simulink model "EV_lunwen_mohu"  (R2018a)
settings: Solver=VariableStepAuto  StartTime=0.0  StopTime=1370  RelTol=1e-3
undefined symbols (not defined in the file or in its folder): batt, cyc_spd, cyc_time, DiscIntNeverNeededParam, fr_effi, TIME_STEP, tm, UC, vcu, vehicle
libraries: simulink x10, fuzblock x1
(part 2 of 2)

== system EV_lunwen_mohu/Vehicle/Fj ==
  veh_spd_mps : Inport
  Dead Zone : DeadZone  LowerValue=-0.01  UpperValue=0.01  SaturateOnIntegerOverflow=on
  Discrete Derivative : simulink/Discrete/Discrete Derivative  gainval=1.0  ICPrevScaledInput=0.0  InputProcessing=Inherited  OutMin=[]  OutMax=[]  OutDataType=fixdt(1, 16)  OutScaling=2^-10  DoSatur=off
  Product1 : Product  SaturateOnIntegerOverflow=on  InputSameDT=on  OutDataTypeStr=Inherit: Same as first input
  Product4 : Product  Inputs=3
  m : Constant  Value=vehicle.veh_mass_kg
  sign(u) : Lookup  InputValues=[ -0.1 0.1 ]  Table="[-1  1]"  LookUpMeth=Interpolation-Use End Values  OutDataTypeStr=double  SaturateOnIntegerOverflow=on
  旋转质量换算系数 : Constant
  Fj : Outport  InitialOutput=0
  wires:
  veh_spd_mps/1 -> Dead Zone/1, Discrete Derivative/1
  Discrete Derivative/1 -> Product4/2
  旋转质量换算系数/1 -> Product4/3
  m/1 -> Product4/1
  sign(u)/1 -> Product1/1
  Dead Zone/1 -> sign(u)/1
  Product4/1 -> Product1/2
  Product1/1 -> Fj/1

== system EV_lunwen_mohu/Vehicle/Fw ==
  veh_spd_mps : Inport
  Dead Zone : DeadZone  LowerValue=-0.01  UpperValue=0.01  SaturateOnIntegerOverflow=on
  Dead Zone1 : DeadZone  LowerValue=-0.01  UpperValue=0.01  SaturateOnIntegerOverflow=on
  Product1 : Product  SaturateOnIntegerOverflow=on  InputSameDT=on  OutDataTypeStr=Inherit: Same as first input
  Product2 : Product  SaturateOnIntegerOverflow=on  InputSameDT=on  OutDataTypeStr=Inherit: Same as first input
  Wind Resistane : Gain  Gain=0.5*vehicle.air_density_kgpm3*vehicle.Cd*vehicle.veh_fac_area_m2  SaturateOnIntegerOverflow=on  OutDataTypeStr=Inherit: Same as input  ParamDataTypeStr=Inherit: Same as input
  sign(u) : Lookup  InputValues=[ -0.1 0.1 ]  Table="[-1  1]"  LookUpMeth=Interpolation-Use End Values  OutDataTypeStr=double  SaturateOnIntegerOverflow=on
  Fi : Outport  InitialOutput=0
  wires:
  Product1/1 -> Wind Resistane/1
  veh_spd_mps/1 -> Dead Zone1/1, Dead Zone/1
  Dead Zone/1 -> Product1/2, Product1/1
  sign(u)/1 -> Product2/1
  Dead Zone1/1 -> sign(u)/1
  Wind Resistane/1 -> Product2/2
  Product2/1 -> Fi/1

== system EV_lunwen_mohu/Vehicle/inertia ==
  inertia_in : Inport
  Product6 : Product  Inputs=3  OutDataTypeStr=double  SaturateOnIntegerOverflow=on  InputSameDT=on
  Sum2 : Sum  Inputs=+++  OutDataTypeStr=double  SaturateOnIntegerOverflow=on
  Tyre radius (m) : Constant  Value=vehicle.tyre_radius_m
  Tyre radius (m)1 : Constant  Value=vehicle.tyre_inertia
  Vehicle mass (kg) : Constant  Value=vehicle.veh_mass_kg
  rad/s^2 to m/s^2 1 : Gain  Gain=4  SaturateOnIntegerOverflow=on  OutDataTypeStr=Inherit: Same as input  ParamDataTypeStr=Inherit: Same as input
  rad/s^2 to m/s^2 2 : Gain  Gain=vehicle.fr_ratio * vehicle.fr_ratio  SaturateOnIntegerOverflow=on  OutDataTypeStr=Inherit: Same as input  ParamDataTypeStr=Inherit: Same as input
  Inertia coefficient : Outport  InitialOutput=0
  wires:
  Tyre radius (m)1/1 -> rad/s^2 to m/s^2 1/1
  Tyre radius (m)/1 -> Product6/3, Product6/2
  Vehicle mass (kg)/1 -> Product6/1
  inertia_in/1 -> rad/s^2 to m/s^2 2/1  "tm_Inertia"
  rad/s^2 to m/s^2 2/1 -> Sum2/1
  Product6/1 -> Sum2/2
  rad/s^2 to m/s^2 1/1 -> Sum2/3
  Sum2/1 -> Inertia coefficient/1

== system EV_lunwen_mohu/BATT/max power limitation/peak chrg power ==
  note: 电池电流
  note: 损耗电压
  note: 电池端电压
  batt_res_ohms : Inport
  batt_oc_volt_v : Inport  Port=2
  Constant : Constant  Value=batt.cell_max_volt_v * batt.cells_series_no
  Constant1 : Constant  Value=0
  Divide : Product  Inputs=*/
  Gain1 : Gain  Gain=1/1000
  MinMax1 : MinMax  Inputs=2  SaturateOnIntegerOverflow=on  InputSameDT=on
  Product2 : Product  SaturateOnIntegerOverflow=on  OutDataTypeStr=Inherit: Same as first input
  Sum1 : Sum  Inputs=+-  SaturateOnIntegerOverflow=on  InputSameDT=on  OutDataTypeStr=Inherit: Same as first input
  chrg_peak_pwr_kw : Outport
  wires:
  Gain1/1 -> chrg_peak_pwr_kw/1
  MinMax1/1 -> Gain1/1
  Constant1/1 -> MinMax1/2
  Product2/1 -> MinMax1/1
  Divide/1 -> Product2/1
  batt_res_ohms/1 -> Divide/2
  Sum1/1 -> Divide/1
  Constant/1 -> Product2/2, Sum1/2
  batt_oc_volt_v/1 -> Sum1/1

== system EV_lunwen_mohu/BATT/max power limitation/peak dischrg power ==
  batt_res_ohms : Inport
  batt_oc_volt_v : Inport  Port=2
  Constant : Constant  Value=batt.cell_min_volt_v * batt.cells_series_no
  Constant1 : Constant  Value=0
  Divide : Product  Inputs=*/
  Gain1 : Gain  Gain=1/1000
  MinMax1 : MinMax  Function=max  Inputs=2  SaturateOnIntegerOverflow=on  InputSameDT=on
  Product2 : Product  SaturateOnIntegerOverflow=on  OutDataTypeStr=Inherit: Same as first input
  Sum1 : Sum  Inputs=+-  SaturateOnIntegerOverflow=on  InputSameDT=on  OutDataTypeStr=Inherit: Same as first input
  dischrg_peak_pwr_kw : Outport
  wires:
  Gain1/1 -> dischrg_peak_pwr_kw/1
  MinMax1/1 -> Gain1/1
  Constant1/1 -> MinMax1/2
  Product2/1 -> MinMax1/1
  Divide/1 -> Product2/1
  batt_res_ohms/1 -> Divide/2
  Sum1/1 -> Divide/1
  Constant/1 -> Product2/2, Sum1/2
  batt_oc_volt_v/1 -> Sum1/1

== system EV_lunwen_mohu/UC and dc//dc/UC/Internal Heating ==
  amb_temp_degc : Inport
  Iout : Inport  Port=2
  lost_volt_v : Inport  Port=3
  1/thermal capacity : Gain  Gain=1/(batt.thermal_capa_jpk*UC.ess_parallel_mod_num*UC.ess_module_num)  SaturateOnIntegerOverflow=on  OutDataTypeStr=Inherit: Same as input  ParamDataTypeStr=Inherit: Same as input
  1/thermal resistance : Gain  Gain=batt.thermal_disp_wpk  SaturateOnIntegerOverflow=on  OutDataTypeStr=Inherit: Same as input  ParamDataTypeStr=Inherit: Same as input
  Abs : Abs  SaturateOnIntegerOverflow=on
  Discrete-Time Integrator1 : DiscreteIntegrator  SampleTime=0.01  LimitOutput=on  LowerSaturationLimit=0  ICPrevOutput=DiscIntNeverNeededParam  ICPrevScaledInput=DiscIntNeverNeededParam
  Product1 : Product  SaturateOnIntegerOverflow=on  InputSameDT=on  OutDataTypeStr=Inherit: Same as first input
  Sum1 : Sum  Inputs=+-  SaturateOnIntegerOverflow=on  InputSameDT=on  OutDataTypeStr=Inherit: Same as first input
  Sum2 : Sum  Inputs=+-  SaturateOnIntegerOverflow=on  InputSameDT=on  OutDataTypeStr=Inherit: Same as first input
  To Workspace : ToWorkspace  VariableName=ess_temp_degc  SaveFormat=Timeseries  SampleTime=-1
  ess_temp_degc : Outport  InitialOutput=0
  wires:
  Sum2/1 -> 1/thermal resistance/1
  amb_temp_degc/1 -> Sum2/2
  Product1/1 -> Abs/1
  Abs/1 -> Sum1/1
  Sum1/1 -> 1/thermal capacity/1
  1/thermal resistance/1 -> Sum1/2
  Iout/1 -> Product1/1
  lost_volt_v/1 -> Product1/2
  1/thermal capacity/1 -> Discrete-Time Integrator1/1
  Discrete-Time Integrator1/1 -> To Workspace/1, ess_temp_degc/1, Sum2/1

== system EV_lunwen_mohu/UC and dc//dc/UC/Subsystem ==
  Preq : Inport
  Voc : Inport  Port=2
  tmp : Inport  Port=3
  SOC : Inport  Port=4
  " " : Fcn  Expr=(u(1)/(u(2)+eps))
  -1*|u| : Fcn  Expr=-1*abs(u)
  Abs : Abs  SaturateOnIntegerOverflow=on
  Delay : Delay  DelayLength=1  InitialCondition=0
  Delay1 : Delay  DelayLength=1  InitialCondition=0
  Iout=(Voc-(Voc^2-4RPout)^.5) ----------------------------- (2*R) : Fcn  Expr=(u[2]-(((u[2]^2-4*u[1]*u[3])>0)*(u[2]^2-4*u[1]*u[3]))^.5)/(2*u[3])
  Memory2 : Memory
  Mux1 : Mux  Inputs=2
  Mux2 : Mux  Inputs=3
  Parallel : Gain  Gain=1/UC.ess_parallel_mod_num  SaturateOnIntegerOverflow=on  OutDataTypeStr=Inherit: Same as input  ParamDataTypeStr=Inherit: Same as input
  Parallel1 : Gain  Gain=1/UC.ess_parallel_mod_num  SaturateOnIntegerOverflow=on  OutDataTypeStr=Inherit: Same as input  ParamDataTypeStr=Inherit: Same as input
  Rchg (ohms) : Lookup2D  RowIndex=UC.ess_tmp  ColumnIndex=UC.ess_i  Table=UC.ess_r  SaturateOnIntegerOverflow=on  InputSameDT=on
  Rdis (ohms) : Lookup2D  RowIndex=UC.ess_tmp  ColumnIndex=UC.ess_i  Table=UC.ess_r  SaturateOnIntegerOverflow=on  InputSameDT=on
  SOClimit : Subsystem
  Subsystem : Subsystem
  Switch2 : Switch  SaturateOnIntegerOverflow=on  InputSameDT=on
  mod # : Gain  Gain=UC.ess_module_num  SaturateOnIntegerOverflow=on  OutDataTypeStr=Inherit: Same as input  ParamDataTypeStr=Inherit: Same as input
  Iout : Outport
  Voc*k : Outport  Port=2
  Rs : Outport  Port=3
  tag scope: ess_max_chg_pwr=global, ess_max_dchg_pwr=global
  wires:
  tmp/1 -> Rchg (ohms)/1, Rdis (ohms)/1
  Mux2/1 -> Iout=(Voc-(Voc^2-4RPout)^.5) ----------------------------- (2*R)/1
  Voc/1 -> mod #/1
  " "/1 -> Abs/1, -1*|u|/1, Switch2/2
  Subsystem/1(Iout_lim) -> Iout/1
  Switch2/1 -> Rs/1, Mux2/3
  Abs/1 -> Rdis (ohms)/2
  Rchg (ohms)/1 -> Parallel/1
  SOClimit/1("Pbty, limited") -> Mux2/1
  Subsystem/2(mx chg pwr) -> Memory2/1
  Memory2/1 -> [ess_max_chg_pwr]
  Iout=(Voc-(Voc^2-4RPout)^.5) ----------------------------- (2*R)/1 -> Subsystem/1(Iout1)
  mod #/1 -> Mux1/2, Subsystem/2(Voc1), Voc*k/1, Mux2/2
  Parallel/1 -> Subsystem/3(Rchg), Switch2/3
  Parallel1/1 -> Switch2/1, Subsystem/4(Rdchg)
  Subsystem/3(mx dchg pwr) -> [ess_max_dchg_pwr]
  SOC/1 -> SOClimit/1(SOC1)
  Preq/1 -> Mux1/1, SOClimit/2(Pbty)
  Mux1/1 -> " "/1
  Delay/1 -> Rchg (ohms)/2
  -1*|u|/1 -> Delay/1
  Delay1/1 -> Parallel1/1
  Rdis (ohms)/1 -> Delay1/1

== system EV_lunwen_mohu/UC and dc//dc/UC/Subsystem1 ==
  Iout : Inport
  C : Inport  Port=2
  Clock : Clock
  Gain : Gain  Gain=UC.ess_parallel_mod_num  SaturateOnIntegerOverflow=on  OutDataTypeStr=Inherit: Same as input  ParamDataTypeStr=Inherit: Same as input
  Memory1 : Memory
  Mux2 : Mux  Inputs=3
  Saturation : Saturate  UpperLimit=1  LowerLimit=0
  Soc = (Voc(n+1)-Vmin)/(Vmax-Vmin) : Fcn  Expr=(u(1)-UC.ess_min_volts)/(UC.ess_max_volts-UC.ess_min_volts)
  Sum : Sum  Inputs=|+-  SaturateOnIntegerOverflow=on  InputSameDT=on  OutDataTypeStr=Inherit: Same as first input
  Voc (n+1) = Voc(n) - I*(dt)/C : Fcn  Expr=(u(1)*u(3)/u(2))
  SOC : Outport
  VOC : Outport  Port=2
  wires:
  Iout/1 -> Mux2/1
  C/1 -> Gain/1
  Soc = (Voc(n+1)-Vmin)/(Vmax-Vmin)/1 -> Saturation/1
  Clock/1 -> Sum/1, Memory1/1
  Mux2/1 -> Voc (n+1) = Voc(n) - I*(dt)/C/1
  Voc (n+1) = Voc(n) - I*(dt)/C/1 -> VOC/1, Soc = (Voc(n+1)-Vmin)/(Vmax-Vmin)/1
  Gain/1 -> Mux2/2
  Sum/1 -> Mux2/3
  Saturation/1 -> SOC/1
  Memory1/1 -> Sum/2

== system EV_lunwen_mohu/VCU/Subsystem1/1st Order Filter ==
  in : Inport
  tc_s : Inport  Port=2
  ts_s : Inport  Port=3
  reset : Inport  Port=4
  Add : Sum
  Add1 : Sum
  Add2 : Sum  Inputs=+-
  Constant : Constant  OutDataTypeStr=single
  Divide : Product  Inputs=*/
  Product : Product  RndMeth=Zero
  Product1 : Product  RndMeth=Zero
  Switch : Switch  Criteria=u2 ~= 0  Threshold=0.5
  Unit Delay : UnitDelay  SampleTime=-1
  out : Outport
  wires:
  Add/1 -> Switch/3
  Product1/1 -> Add/2
  Product/1 -> Add/1
  Add2/1 -> Product/2
  in/1 -> Product/1, Switch/1
  Divide/1 -> Product1/1, Add2/2
  Constant/1 -> Add2/1
  Add1/1 -> Divide/2
  ts_s/1 -> Add1/2
  tc_s/1 -> Divide/1, Add1/1
  Unit Delay/1 -> Product1/2
  reset/1 -> Switch/2
  Switch/1 -> out/1, Unit Delay/1

== system EV_lunwen_mohu/VCU/Subsystem3/RateLimit ==
  note: 单位时间内力矩输出（力矩转换速率）
  note: 单位时间内力矩输出的变化量应在转换速率区间内
  note: -10000
  note: 10000
  in : Inport  PortDimensions=1
  steptime : Inport  Port=2  PortDimensions=1
  ratelimt_inc : Inport  Port=3  PortDimensions=1
  ratelimt_dec : Inport  Port=4  PortDimensions=1
  MinMax : MinMax  Inputs=2
  MinMax1 : MinMax  Function=max  Inputs=2
  MinMax2 : MinMax  Function=max  Inputs=2
  MinMax3 : MinMax  Inputs=2
  Product : Product  RndMeth=Zero
  Product1 : Product  RndMeth=Zero
  Sum5 : Sum  Inputs=+-
  Sum6 : Sum
  UnitDelay1 : UnitDelay  SampleTime=-1
  step_time6 : Constant  Value=0  OutDataTypeStr=single
  out : Outport
  wires:
  ratelimt_inc/1 -> Product/1
  MinMax3/1 -> [Dec]
  MinMax2/1 -> [Inc]
  step_time6/1 -> MinMax3/1, MinMax2/2
  Product1/1 -> MinMax3/2
  Product/1 -> MinMax2/1
  UnitDelay1/1 -> Sum6/2, Sum5/2
  Sum6/1 -> UnitDelay1/1, out/1
  in/1 -> Sum5/1
  MinMax/1 -> Sum6/1
  MinMax1/1 -> MinMax/2
  [Inc] -> MinMax/1
  [Dec] -> MinMax1/2
  Sum5/1 -> MinMax1/1
  steptime/1 -> Product/2, Product1/1
  ratelimt_dec/1 -> Product1/2

== system EV_lunwen_mohu/VCU/续驶里程估计/Subsystem ==
  VehicleSpeed : Inport
  BattVlt : Inport  Port=2
  BattCurr : Inport  Port=3
  BattSOC : Inport  Port=4
  Add : Sum  Inputs=+-
  Chart1 : Stateflow chart  TreatAsAtomicUnit=on
  Constant14 : Constant  Value=80  OutDataTypeStr=double
  Discrete-Time Integrator : DiscreteIntegrator  SampleTime=0.01  OutDataTypeStr=double  ICPrevOutput=DiscIntNeverNeededParam  ICPrevScaledInput=DiscIntNeverNeededParam
  Discrete-Time Integrator2 : DiscreteIntegrator  SampleTime=0.01  OutDataTypeStr=double  ICPrevOutput=DiscIntNeverNeededParam  ICPrevScaledInput=DiscIntNeverNeededParam
  Gain : Gain  Gain=1/3600  OutDataTypeStr=double
  Gain1 : Gain  Gain=1/3600000  OutDataTypeStr=double
  Gain2 : Gain  Gain=1.6093  OutDataTypeStr=double
  Gain4 : Gain  Gain=1/1000  OutDataTypeStr=double
  Product4 : Product  OutDataTypeStr=single
  Scope1 : Scope
  Scope2 : Scope
  Scope3 : Scope
  To Workspace : ToWorkspace  VariableName=sp  SaveFormat=Timeseries  SampleTime=-1
  To Workspace1 : ToWorkspace  VariableName=Ecost1  SampleTime=-1
  To Workspace2 : ToWorkspace  VariableName=S11  SampleTime=-1
  Unit Delay1 : UnitDelay  SampleTime=-1
  wires:
  Discrete-Time Integrator/1 -> Gain/1
  VehicleSpeed/1 -> Gain2/1
  Product4/1 -> Discrete-Time Integrator2/1
  Discrete-Time Integrator2/1 -> Gain1/1
  BattCurr/1 -> Product4/2
  Gain1/1 -> Chart1/7(Ei)
  BattVlt/1 -> Gain4/1, Product4/1
  Gain4/1 -> Chart1/5(U)
  BattSOC/1 -> Chart1/4(SOC)
  Constant14/1 -> Chart1/6(C)
  Unit Delay1/1 -> Add/2
  Add/1 -> Chart1/3(DetaV)
  Gain/1 -> Scope3/1, Chart1/2(S)
  Chart1/1(JL) -> To Workspace/1, Scope1/1
  Gain2/1 -> Add/1, Scope2/1, Chart1/1(v), Discrete-Time Integrator/1, Unit Delay1/1
  Chart1/3(S1) -> To Workspace2/1
  Chart1/2(Ecost) -> To Workspace1/1

== system EV_lunwen_mohu/UC and dc//dc/UC/Subsystem/SOClimit ==
  SOC1 : Inport
  Pbty : Inport  Port=2
  Constant1 : Constant  Value=0.001
  Constant5 : Constant  Value=.999
  Constant9 : Constant  Value=0
  Logical Operator : Logic  Operator=OR
  Logical Operator1 : Logic
  Logical Operator2 : Logic  Operator=NOT  Inputs=1
  Relational Operator : RelationalOperator  Operator=>  RndMeth=Nearest  InputSameDT=on
  Relational Operator3 : RelationalOperator  Operator=<  RndMeth=Nearest  InputSameDT=on
  SOC>=.999 : RelationalOperator  RndMeth=Nearest  InputSameDT=on
  charging (Preq is neg) : RelationalOperator  Operator=<  RndMeth=Nearest  InputSameDT=on
  no power req if SOC<0 and trying to discharge : Switch  Threshold=eps  SaturateOnIntegerOverflow=on  InputSameDT=on
  no power req if SOC>.999 and trying to charge : Switch  Threshold=eps  SaturateOnIntegerOverflow=on  InputSameDT=on
  "Pbty, limited" : Outport  InitialOutput=0
  tag scope: ess_soc_hi_limited=global, ess_soc_low_limited=global
  wires:
  Constant9/1 -> charging (Preq is neg)/2, Relational Operator3/2, no power req if SOC>.999 and trying to charge/1, no power req if SOC<0 and trying to discharge/3
  Logical Operator1/1 -> no power req if SOC>.999 and trying to charge/2, [ess_soc_hi_limited]
  SOC>=.999/1 -> Logical Operator1/1
  no power req if SOC>.999 and trying to charge/1 -> "Pbty, limited"/1
  Logical Operator/1 -> no power req if SOC<0 and trying to discharge/2, Logical Operator2/1
  Constant1/1 -> Relational Operator/2
  Constant5/1 -> SOC>=.999/2
  SOC1/1 -> SOC>=.999/1, Relational Operator/1
  no power req if SOC<0 and trying to discharge/1 -> no power req if SOC>.999 and trying to charge/3
  Relational Operator/1 -> Logical Operator/1
  Pbty/1 -> no power req if SOC<0 and trying to discharge/1, charging (Preq is neg)/1, Relational Operator3/1
  Relational Operator3/1 -> Logical Operator/2
  Logical Operator2/1 -> [ess_soc_low_limited]
  charging (Preq is neg)/1 -> Logical Operator1/2

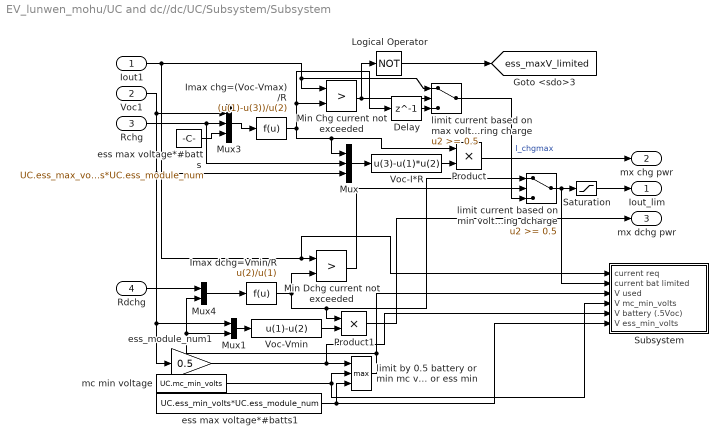
== system EV_lunwen_mohu/UC and dc//dc/UC/Subsystem/Subsystem ==
  Iout1 : Inport
  Voc1 : Inport  Port=2
  Rchg : Inport  Port=3
  Rdchg : Inport  Port=4
  Delay : Delay  DelayLength=1  InitialCondition=0
  Imax chg=(Voc-Vmax)/R : Fcn  Expr=(u(1)-u(3))/u(2)
  Imax dchg=Vmin/R : Fcn  Expr=u(2)/u(1)
  Logical Operator : Logic  Operator=NOT
  Min Chg current not exceeded : RelationalOperator  Operator=>  RndMeth=Nearest  InputSameDT=on
  Min Dchg current not exceeded : RelationalOperator  Operator=>  RndMeth=Nearest  InputSameDT=on
  Mux : Mux  Inputs=3
  Mux1 : Mux  Inputs=2
  Mux3 : Mux  Inputs=3
  Mux4 : Mux  Inputs=2
  Product : Product  SaturateOnIntegerOverflow=on  RndMeth=Zero  InputSameDT=on  OutDataTypeStr=Inherit: Same as first input
  Product1 : Product  SaturateOnIntegerOverflow=on  RndMeth=Zero  InputSameDT=on  OutDataTypeStr=Inherit: Same as first input
  Saturation : Saturate  UpperLimit=2000*UC.ess_parallel_mod_num  LowerLimit=-2000*UC.ess_parallel_mod_num
  Subsystem : Subsystem
  Voc-I*R : Fcn  Expr=u(3)-u(1)*u(2)
  Voc-Vmin : Fcn  Expr=u(1)-u(2)
  ess max voltage*#batts : Constant  Value=UC.ess_max_volts*UC.ess_module_num
  ess max voltage*#batts1 : Constant  Value=UC.ess_min_volts*UC.ess_module_num
  ess_module_num1 : Gain  Gain=0.5  SaturateOnIntegerOverflow=on  OutDataTypeStr=Inherit: Same as input  ParamDataTypeStr=Inherit: Same as input
  limit by 0.5 battery or min mc voltage or ess min : MinMax  Function=max  Inputs=3  SaturateOnIntegerOverflow=on  InputSameDT=on
  limit current based on max voltage during charge : Switch  Threshold=0.5  SaturateOnIntegerOverflow=on  InputSameDT=on
  limit current based on min voltage during dcharge : Switch  Threshold=0.5  SaturateOnIntegerOverflow=on  InputSameDT=on
  mc min voltage : Constant  Value=UC.mc_min_volts
  Iout_lim : Outport
  mx chg pwr : Outport  Port=2
  mx dchg pwr : Outport  Port=3
  tag scope: ess_maxV_limited=global
  wires:
  Product1/1 -> mx dchg pwr/1
  Imax chg=(Voc-Vmax)/R/1 -> Product/1, Mux/1, Delay/1, Min Chg current not exceeded/2
  Imax dchg=Vmin/R/1 -> limit current based on min voltage during dcharge/1, Product1/1, Min Dchg current not exceeded/2
  Voc-I*R/1 -> Product/2
  Mux3/1 -> Imax chg=(Voc-Vmax)/R/1
  Voc1/1 -> Mux1/1, ess_module_num1/1, Mux/3, Mux3/1
  Min Chg current not exceeded/1 -> Logical Operator/1, limit current based on max voltage during charge/2
  Rchg/1 -> Mux/2, Mux3/2
  ess max voltage*#batts/1 -> Mux3/3
  Min Dchg current not exceeded/1 -> limit current based on min voltage during dcharge/2
  Mux4/1 -> Imax dchg=Vmin/R/1
  limit current based on max voltage during charge/1 -> limit current based on min voltage during dcharge/3  "I_chgmax"
  Rdchg/1 -> Mux4/1
  Logical Operator/1 -> [ess_maxV_limited]
  Saturation/1 -> Iout_lim/1
  Mux/1 -> Voc-I*R/1
  Product/1 -> mx chg pwr/1
  Voc-Vmin/1 -> Product1/2
  Mux1/1 -> Voc-Vmin/1
  Iout1/1 -> Subsystem/1(current req), Min Dchg current not exceeded/1, limit current based on max voltage during charge/1, Min Chg current not exceeded/1
  limit current based on min voltage during dcharge/1 -> Saturation/1, Subsystem/2(current bat limited)
  limit by 0.5 battery or min mc voltage or ess min/1 -> Subsystem/3(V used), Mux1/2, Mux4/2
  mc min voltage/1 -> Subsystem/4(V mc_min_volts), limit by 0.5 battery or min mc voltage or ess min/2
  ess_module_num1/1 -> Subsystem/5(V battery (.5Voc)), limit by 0.5 battery or min mc voltage or ess min/1
  ess max voltage*#batts1/1 -> Subsystem/6(V ess_min_volts), limit by 0.5 battery or min mc voltage or ess min/3
  Delay/1 -> limit current based on max voltage during charge/3

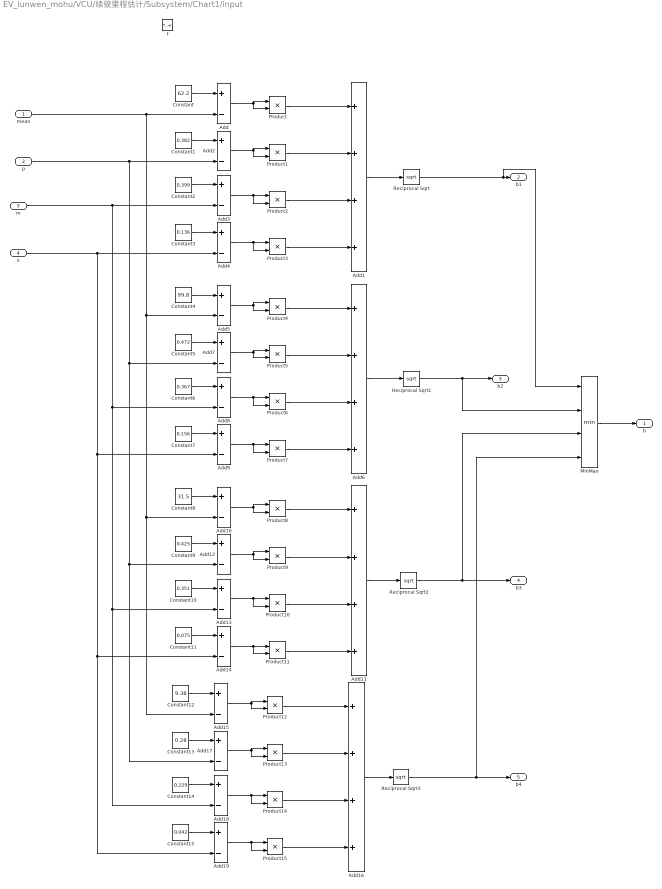
== system EV_lunwen_mohu/VCU/续驶里程估计/Subsystem/Chart1/input ==
  mean : Inport  OutDataTypeStr=double  PortDimensions=1
  p : Inport  Port=2  OutDataTypeStr=double  PortDimensions=1
  m : Inport  Port=3  OutDataTypeStr=double  PortDimensions=1
  n : Inport  Port=4  OutDataTypeStr=double  PortDimensions=1
  f : TriggerPort  TriggerType=function-call  VariantControl=Variant
      settings: CopyFcn=Stateflow.SLINSF.SimulinkMan.removeBlockPreDeleteFcn  PreDeleteFcn=Stateflow.SLINSF.SimulinkMan.unsafePredeleteFcn
  Add{,2..5,7..10,12..15,17..19} (16 alike) : Sum  Inputs=+-
  Add{1,6,11,16} (4 alike) : Sum  Inputs=++++
  Constant : Constant  Value=62.2
  Constant1 : Constant  Value=0.382
  Constant10 : Constant  Value=0.351
  Constant11 : Constant  Value=0.075
  Constant12 : Constant  Value=9.38
  Constant13 : Constant  Value=0.28
  Constant14 : Constant  Value=0.229
  Constant15 : Constant  Value=0.042
  Constant2 : Constant  Value=0.399
  Constant3 : Constant  Value=0.136
  Constant4 : Constant  Value=99.8
  Constant5 : Constant  Value=0.472
  Constant6 : Constant  Value=0.367
  Constant7 : Constant  Value=0.156
  Constant8 : Constant  Value=31.5
  Constant9 : Constant  Value=0.425
  MinMax : MinMax  Inputs=4
  Product{,1..15} (16 alike) : Product
  Reciprocal Sqrt{,1..3} (4 alike) : Sqrt  SaturateOnIntegerOverflow=on
  b : Outport
  b1 : Outport  Port=2
  b2 : Outport  Port=3
  b3 : Outport  Port=4
  b4 : Outport  Port=5
  wires:
  MinMax/1 -> b/1
  Constant/1 -> Add/1
  mean/1 -> Add/2, Add15/2, Add10/2, Add5/2
  Add/1 -> Product/1, Product/2
  Constant1/1 -> Add2/1
  p/1 -> Add17/2, Add12/2, Add7/2, Add2/2
  Add2/1 -> Product1/1, Product1/2
  Constant2/1 -> Add3/1
  m/1 -> Add18/2, Add13/2, Add8/2, Add3/2
  Add3/1 -> Product2/2, Product2/1
  Constant3/1 -> Add4/1
  n/1 -> Add19/2, Add14/2, Add9/2, Add4/2
  Add4/1 -> Product3/2, Product3/1
  Add1/1 -> Reciprocal Sqrt/1
  Product/1 -> Add1/1
  Product1/1 -> Add1/2
  Product2/1 -> Add1/3
  Product3/1 -> Add1/4
  Constant4/1 -> Add5/1
  Add5/1 -> Product4/1, Product4/2
  Constant5/1 -> Add7/1
  Add7/1 -> Product5/1, Product5/2
  Constant6/1 -> Add8/1
  Add8/1 -> Product6/2, Product6/1
  Constant7/1 -> Add9/1
  Add9/1 -> Product7/2, Product7/1
  Add6/1 -> Reciprocal Sqrt1/1
  Product4/1 -> Add6/1
  Product5/1 -> Add6/2
  Product6/1 -> Add6/3
  Product7/1 -> Add6/4
  Constant8/1 -> Add10/1
  Add10/1 -> Product8/1, Product8/2
  Constant9/1 -> Add12/1
  Add12/1 -> Product9/1, Product9/2
  Constant10/1 -> Add13/1
  Add13/1 -> Product10/2, Product10/1
  Constant11/1 -> Add14/1
  Add14/1 -> Product11/2, Product11/1
  Add11/1 -> Reciprocal Sqrt2/1
  Product8/1 -> Add11/1
  Product9/1 -> Add11/2
  Product10/1 -> Add11/3
  Product11/1 -> Add11/4
  Constant12/1 -> Add15/1
  Add15/1 -> Product12/1, Product12/2
  Constant13/1 -> Add17/1
  Add17/1 -> Product13/1, Product13/2
  Constant14/1 -> Add18/1
  Add18/1 -> Product14/2, Product14/1
  Constant15/1 -> Add19/1
  Add19/1 -> Product15/2, Product15/1
  Add16/1 -> Reciprocal Sqrt3/1
  Product12/1 -> Add16/1
  Product13/1 -> Add16/2
  Product14/1 -> Add16/3
  Product15/1 -> Add16/4
  Reciprocal Sqrt1/1 -> b2/1, MinMax/2
  Reciprocal Sqrt/1 -> b1/1, MinMax/1
  Reciprocal Sqrt2/1 -> b3/1, MinMax/3
  Reciprocal Sqrt3/1 -> b4/1, MinMax/4

== system EV_lunwen_mohu/UC and dc//dc/UC/Subsystem/Subsystem/Subsystem ==
  current req : Inport
  current bat limited : Inport  Port=2
  V used : Inport  Port=3
  V mc_min_volts : Inport  Port=4
  V battery (.5Voc) : Inport  Port=5
  V ess_min_volts : Inport  Port=6
  Relational Operator1 : RelationalOperator  Operator===  RndMeth=Nearest  InputSameDT=on
  Relational Operator3 : RelationalOperator  Operator===  RndMeth=Nearest  InputSameDT=on
  Relational Operator4 : RelationalOperator  Operator===  RndMeth=Nearest  InputSameDT=on
  Relational Operator5 : RelationalOperator  Operator=<=  RndMeth=Nearest  InputSameDT=on
  limited by battery : Logic
  limited by battery min V : Logic
  limited by motor controller : Logic
  tag scope: ess_minV_limited=global, ess_pwr_limited=global, mc_voltage_limited=global
  wires:
  Relational Operator1/1 -> limited by battery min V/1, limited by battery/1, limited by motor controller/1
  V used/1 -> Relational Operator5/1, Relational Operator4/1, Relational Operator3/1
  Relational Operator4/1 -> limited by battery/2
  Relational Operator5/1 -> limited by battery min V/2
  Relational Operator3/1 -> limited by motor controller/2
  V ess_min_volts/1 -> Relational Operator5/2
  V mc_min_volts/1 -> Relational Operator3/2
  current bat limited/1 -> Relational Operator1/2
  limited by battery/1 -> [ess_pwr_limited]
  current req/1 -> Relational Operator1/1
  limited by battery min V/1 -> [ess_minV_limited]
  V battery (.5Voc)/1 -> Relational Operator4/2
  limited by motor controller/1 -> [mc_voltage_limited]

== stateflow chart EV_lunwen_mohu/VCU/续驶里程估计/Subsystem/Chart1 ==
  state cul
    state run
      du:
      sumv=sumv+v;
      LL=S/Ei;
      if  (DetaV>0)
      i = i + 1;
      elseif (DetaV==0&&v~=0)
      j=j+1;
      elseif(DetaV<0)
      k=k+1;
      end
    state choose
      en:meanv=sumv/6000,P=i/6000,M=j/6000,N=k/6000;
      [d,d1,d2,d3,d4]=input(meanv,P,M,N);
      if(d==d1)
      E=0.3508;
      JL=1;
      elseif(d==d2)
      E=0.6888;
      JL=2;
      elseif(d==d3)
      E=0.141;
      JL=3;
      elseif(d==d4)
      E=0.0789;
      JL=4;
      end
      i=0,j=0,k=0,m=m+1;
      sumv=0;
      E_out=Ei-E_temp;
      LL=(S-S1)/E;
    state cull
      en:
      Ecost=Ecost+E;
      Erest=Etotal-Ecost;
      l=2+0.2066*(Erest-4);
      Srest=l*Erest;
      E_temp=Ei;
      S1=S;
    (default) -> run
    cull -> run
    run -> choose : after(60,sec)
    choose -> cull
  state init
    en:i=0,j=0,k=0,m=0,sumv=0;
    Etotal=U*C*SOC,E_temp=0;
    Ecost=0;Srest_compare=0;
    du:Etotal=U*C*SOC;
    Srest=Etotal*6;
    S1=0;E=0.15;
  state [b,b1,b2,b3,b4]=input(mean,p,m,n) [function]
  init -> cul : after(3,tick)
  (default) -> init
  data: mean function_input double size=1; p function_input double size=1; m function_input double size=1; n function_input double size=1; b function_output; b1 function_output; b2 function_output; b3 function_output; b4 function_output; JL output; v input; S input; DetaV input; i local; j local; k local; sumv local; meanv local; P local; M local; N local; m local; d1 local; d2 local; d3 local; d4 local; d local; E local; Etotal local; SOC input; U input; Srest local; Ecost output; l local; Ecost_temp local; Erest local; Srest_compare local; C input; Ei input; E_out local; E_temp local; LL local; S1 output
